simulink model "Thermocouple_Voltage_generation"  (R2019a)
settings: Solver=ode23t  StartTime=0.0  StopTime=0.5  FixedStep=Ts  MaxStep=1e-4  RelTol=1e-3  EnableMultiTasking=on
PreLoadFcn:
  | ee_inverting_buck_boost_converter_control_data;
StopFcn:
  | ee_addSimlogTimeStamp(bdroot)
undefined symbols (not defined in the file): Ki, Kp, Rload, Ts, Tsc
libraries: fl_lib x8, nesl_utility x7, ee_lib x2, eeDcDcVoltageController x1, eePwmGenerator x1
CloseFcn:
  | try,close(h1_ee_inverting_buck_boost_converter_control),end
  | clear h1_ee_inverting_buck_boost_converter_control
  | 
  | clear simlog_ee_inverting_buck_boost_converter_control
  | clear logsout_ee_inverting_buck_boost_converter_control
Description:
  | Inverting Topology Buck-Boost Converter Control
settings Model: Creator=The MathWorks, Inc.  LastModifiedBy=user
settings DataIOCC: MaxDataPoints=210000  ReturnWorkspaceOutputs=off  SignalLoggingName=logsout_ee_inverting_buck_boost_converter_control
settings OptimizationCC: LifeSpan=inf
settings DebuggingCC: UnderspecifiedInitializationDetection=Classic  MergeDetectMultiDrivingBlocksExec=none  PregeneratedLibrarySubsystemCodeDiagnostic=none  SFUnexpectedBacktrackingDiag=warning  SFNoUnconditionalDefaultTransitionDiag=warning  SFExecutionAtInitializationDiag=none  ArithmeticOperatorsInVariantConditions=warning
settings SFSimCC: SimUseLocalCustomCode=off
settings RTWCC: RTWUseLocalCustomCode=off
settings CodeAppCC: StateflowObjectComments=on
settings GRTTargetCC: TargetLangStandard=C89/C90 (ANSI)  GeneratePreprocessorConditionals=Disable all
settings ConfigComp: CovMetricSettings=dw  CovHtmlReporting=on  CovSaveCumulativeToWorkspaceVar=on  CovSaveSingleToWorkspaceVar=on  CovExternalEMLEnable=off
settings SimscapeCC: SimscapeNormalizeSystem=off  SimscapeLogType=all  SimscapeLogSimulationStatistics=on  SimscapeLogName=simlog_ee_inverting_buck_boost_converter_control  SimscapeLogDataHistory=210000

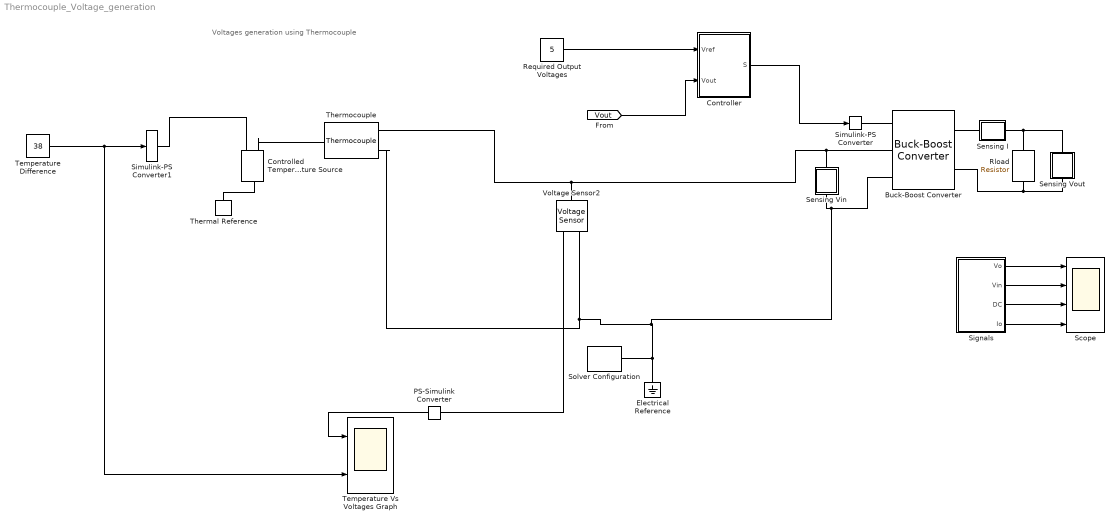
== system Thermocouple_Voltage_generation ==
  note: Voltages generation using Thermocouple
  Buck-Boost Converter : ee_lib/Semiconductors & Converters/Converters/Buck-Boost Converter  device_type=3  Vf=0.8 V  Ron=0.001 Ohm  Rds=1e-9 Ohm  Goff=1e-9 1/Ohm  Vth=0.5 V  Vgt=1 V  Vgt_off=-1 V  Ih=1 A  diode_param=2  diode_Vf=0.8 V  diode_Ron=1e-9 Ohm  diode_Goff=1e-6 1/Ohm  diode_C=50 nF  diode_iRM=-235 A  diode_iF=300 A  diode_idot=-50 A/us  diode_trr_param=1  diode_trr_factor=3  diode_trr=15 us  diode_Qrr=1500 s*uA  Lf=L H  Cf=C F  Rf=R Ohm  snubber_type=1  Rs=0.1 Ohm  Cs=1e-7 F
      settings: SourceProductName=Simscape Electrical  SourceProductBaseCode=PS
  Controlled Temperature Source : fl_lib/Thermal/Thermal Sources/Controlled Temperature Source
      settings: SourceProductName=Simscape
  Controller : Subsystem
  Electrical Reference : fl_lib/Electrical/Electrical Elements/Electrical Reference
  PS-Simulink Converter : nesl_utility/PS-Simulink Converter  PhysicalDomain=network_engine_domain  SubClassName=ps_output  LeftPortType=input  RightPortType=output  PseudoPeriodic=off  Frequencies=[]  Unit=1  AffineConversion=off
  Required Output Voltages : Constant  Value=5
  Rload : fl_lib/Electrical/Electrical Elements/Resistor  R=Rload Ohm  i_specify=off  i_priority=None  i=0 A  i_nominal_specify=off  i_nominal_unit=A  i_nominal_value=1  v_specify=off  v_priority=None  v=0 V  v_nominal_specify=off  v_nominal_unit=V  v_nominal_value=1
  Scope : Scope  NumInputPorts=4
  Sensing Vin : Subsystem
      mask Display:
      | disp('V')
      | port_label('Lconn',1,'+')
      | port_label('Rconn',1,'-')
  Sensing Vout : Subsystem
      mask Display:
      | disp('V')
      | port_label('Lconn',1,'+')
      | port_label('Rconn',1,'-')
  Sensing I : Subsystem
      mask Display:
      | disp('I')
      | port_label('Lconn',1,'+')
      | port_label('Rconn',1,'-')
  Signals : Subsystem
  Simulink-PS Converter : nesl_utility/Simulink-PS Converter  PhysicalDomain=network_engine_domain  SubClassName=ps_input  LeftPortType=input  RightPortType=output  PseudoPeriodic=off  Frequencies=[]  NoiseDistribution=none  NoiseParameters=[]  Unit=1  AffineConversion=off  FilteringAndDerivatives=provide  SimscapeFilterOrder=1  InputFilterTimeConstant=0.001  UdotUserProvided=0
  Simulink-PS Converter1 : nesl_utility/Simulink-PS Converter  PhysicalDomain=network_engine_domain  SubClassName=ps_input  LeftPortType=input  RightPortType=output  PseudoPeriodic=off  Frequencies=[]  NoiseDistribution=none  NoiseParameters=[]  Unit=K  AffineConversion=off  FilteringAndDerivatives=provide  SimscapeFilterOrder=1  InputFilterTimeConstant=0.001  UdotUserProvided=0
  Solver Configuration : nesl_utility/Solver Configuration  PhysicalDomain=network_engine_domain  SubClassName=solver  LeftPortType=input  RightPortType=generic  Tones=[]  Harmonics=[]  SimulateNoise=off  Profile=off  UseLocalSampling=off  EnableSwitchedLinearOptims=on  FrequencyDomain=off  UseCCode=off  RelTol=0.001  AbsTol=1e-06  MinStep=1e-09  ToWorkspace=off  RevertToSquareIcSolve=off  NumHomotopyIterations=100  PhasorMode=off  PhasorModeNumHarmonics=1  DoDC=off  ResidualTolerance=1e-9  UseLocalSolver=on  LocalSolverChoice=NE_BACKWARD_EULER_ADVANCER  LocalSolverSampleTime=Ts  DoFixedCost=on  MaxNonlinIter=3  MaxModeIter=2  LinearAlgebra=auto  EquationFormulation=NE_TIME_EF  DelaysMemoryBudget=1024  AutomaticFiltering=on  FilteringTimeConstant=0.001  PartitionStorageMethod=AS_NEEDED  PartitionMemoryBudget=1024  PartitionMethod=FAST
  "Temperature Difference " : Constant  Value=38
  Temperature Vs Voltages Graph : Scope  NumInputPorts=2
  Thermal Reference : fl_lib/Thermal/Thermal Elements/Thermal Reference
  Thermocouple : ee_lib/Sensors & Transducers/Thermocouple  thermocouple_type=2  Cvec=[1, 1, 0.05, 0, 0, 0, 0, 0, 0]  Avec=[1,0, 0]  T0=0 degC  tc=1 s  K_d=1e-3 W/K  init_temp=25 degC
      settings: SourceProductName=Simscape Electrical  SourceProductBaseCode=PS
  Voltage Sensor2 : fl_lib/Electrical/Electrical Sensors/Voltage Sensor
  wires:
  Required Output Voltages/1 -> Controller/1(Vref)
  Controller/1(S) -> Simulink-PS Converter/1
  [Vout] -> Controller/2(Vout)
  Signals/1(Vo) -> Scope/1
  Signals/3(DC) -> Scope/3
  Signals/4(Io) -> Scope/4
  Signals/2(Vin) -> Scope/2
  PS-Simulink Converter/1 -> Temperature Vs Voltages Graph/1
  "Temperature Difference "/1 -> Simulink-PS Converter1/1, Temperature Vs Voltages Graph/2
  connections:
  Thermocouple/LConn2 -- Voltage Sensor2/RConn2 -- Solver Configuration/RConn1 -- Electrical Reference/LConn1 -- Sensing Vin/RConn1 -- Buck-Boost Converter/LConn3
  Rload/LConn1 -- Sensing Vout/RConn1 -- Sensing I/LConn1
  Buck-Boost Converter/RConn2 -- Rload/RConn1 -- Sensing Vout/LConn1
  Voltage Sensor2/LConn1 -- Thermocouple/LConn1 -- Sensing Vin/LConn1 -- Buck-Boost Converter/LConn2
  Simulink-PS Converter/RConn1 -- Buck-Boost Converter/LConn1
  Sensing I/RConn1 -- Buck-Boost Converter/RConn1
  Simulink-PS Converter1/RConn1 -- Controlled Temperature Source/RConn1
  PS-Simulink Converter/LConn1 -- Voltage Sensor2/RConn1
  Controlled Temperature Source/LConn1 -- Thermal Reference/LConn1
  Controlled Temperature Source/RConn2 -- Thermocouple/RConn1

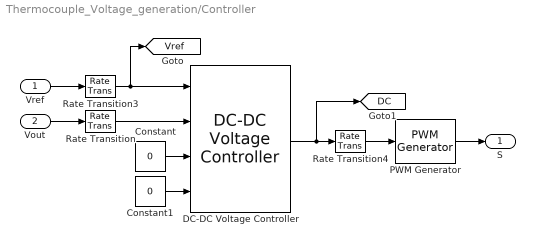
== system Thermocouple_Voltage_generation/Controller ==
  Vref : Inport
  Vout : Inport  Port=2
  Constant : Constant  Value=0
  Constant1 : Constant  Value=0
  DC-DC Voltage Controller : eeDcDcVoltageController/DC-DC Voltage Controller  Kp=Kp  Ki=Ki  Kaw=1  up=0.95  lo=0  Ts=Tsc  Tf=0.001  ActVdcFilter=off
      settings: SourceProductName=Simscape Electrical  SourceProductBaseCode=PS
  PWM Generator : eePwmGenerator/PWM Generator  CarrCount=Up  Tper=1e-4  Ts=Ts
      settings: SourceProductName=Simscape Electrical
  Rate Transition : RateTransition  OutPortSampleTime=Tsc
  Rate Transition3 : RateTransition  OutPortSampleTime=Tsc
  Rate Transition4 : RateTransition  OutPortSampleTime=Ts
  S : Outport
  tag scope: DC=global, Vref=global
  wires:
  Vref/1 -> Rate Transition3/1
  Rate Transition3/1 -> DC-DC Voltage Controller/1, [Vref]
  Vout/1 -> Rate Transition/1
  PWM Generator/1 -> S/1
  DC-DC Voltage Controller/1 -> Rate Transition4/1, [DC]
  Rate Transition4/1 -> PWM Generator/1
  Rate Transition/1 -> DC-DC Voltage Controller/2
  Constant/1 -> DC-DC Voltage Controller/3
  Constant1/1 -> DC-DC Voltage Controller/4

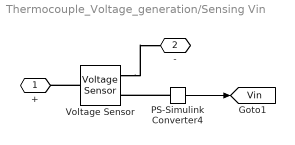
== system Thermocouple_Voltage_generation/Sensing Vin ==
  PS-Simulink Converter4 : nesl_utility/PS-Simulink Converter  PhysicalDomain=network_engine_domain  SubClassName=ps_output  LeftPortType=input  RightPortType=output  PseudoPeriodic=off  Frequencies=[]  Unit=V  AffineConversion=off
  Voltage Sensor : fl_lib/Electrical/Electrical Sensors/Voltage Sensor
  + : PMIOPort  Side=Left
  - : PMIOPort  Port=2  Side=Right
  tag scope: Vin=global
  wires:
  PS-Simulink Converter4/1 -> [Vin]
  connections:
  PS-Simulink Converter4/LConn1 -- Voltage Sensor/RConn1
  Voltage Sensor/RConn2 -- -/RConn1
  Voltage Sensor/LConn1 -- +/RConn1

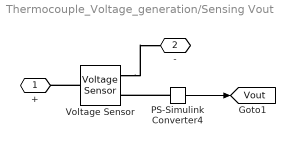
== system Thermocouple_Voltage_generation/Sensing Vout ==
  PS-Simulink Converter4 : nesl_utility/PS-Simulink Converter  PhysicalDomain=network_engine_domain  SubClassName=ps_output  LeftPortType=input  RightPortType=output  PseudoPeriodic=off  Frequencies=[]  Unit=V  AffineConversion=off
  Voltage Sensor : fl_lib/Electrical/Electrical Sensors/Voltage Sensor
  + : PMIOPort  Side=Left
  - : PMIOPort  Port=2  Side=Right
  tag scope: Vout=global
  wires:
  PS-Simulink Converter4/1 -> [Vout]
  connections:
  Voltage Sensor/LConn1 -- +/RConn1
  Voltage Sensor/RConn2 -- -/RConn1
  PS-Simulink Converter4/LConn1 -- Voltage Sensor/RConn1

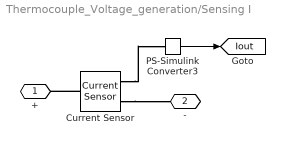
== system Thermocouple_Voltage_generation/Sensing I ==
  Current Sensor : fl_lib/Electrical/Electrical Sensors/Current Sensor
  PS-Simulink Converter3 : nesl_utility/PS-Simulink Converter  PhysicalDomain=network_engine_domain  SubClassName=ps_output  LeftPortType=input  RightPortType=output  PseudoPeriodic=off  Frequencies=[]  Unit=A  AffineConversion=off
  + : PMIOPort  Side=Left
  - : PMIOPort  Port=2  Side=Right
  tag scope: Iout=global
  wires:
  PS-Simulink Converter3/1 -> [Iout]
  connections:
  Current Sensor/RConn1 -- PS-Simulink Converter3/LConn1
  Current Sensor/LConn1 -- +/RConn1
  Current Sensor/RConn2 -- -/RConn1

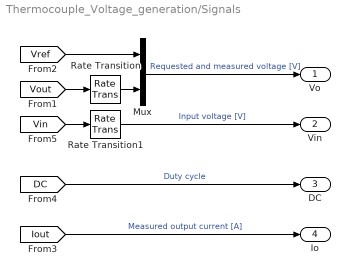
== system Thermocouple_Voltage_generation/Signals ==
  Mux : Mux  Inputs=2
  Rate Transition : RateTransition  OutPortSampleTime=Tsc
  Rate Transition1 : RateTransition  OutPortSampleTime=Tsc
  Vo : Outport
  Vin : Outport  Port=2
  DC : Outport  Port=3
  Io : Outport  Port=4
  wires:
  [Vout] -> Rate Transition/1
  [Vin] -> Rate Transition1/1
  Rate Transition1/1 -> Vin/1  "Input voltage [V]"
  Mux/1 -> Vo/1  "Requested and measured voltage [V]"
  [Iout] -> Io/1  "Measured output current [A]"
  [Vref] -> Mux/1
  Rate Transition/1 -> Mux/2
  [DC] -> DC/1  "Duty cycle"
